simulink model "simplevector"  (R2014a)
settings: Solver=ode45  StartTime=0.0  StopTime=10.0  RelTol=1e-3
settings Model: Creator=RANGA  LastModifiedBy=RANGA

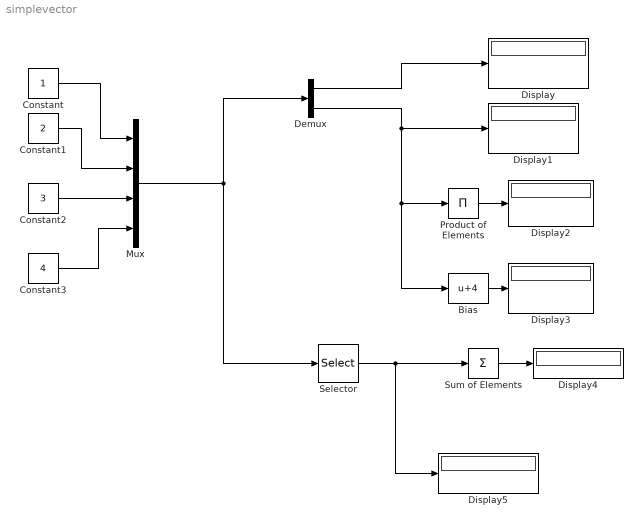
== system simplevector ==
  Bias : Bias  Bias=4
  Constant : Constant
  Constant1 : Constant  Value=2
  Constant2 : Constant  Value=3
  Constant3 : Constant  Value=4
  Demux : Demux  Outputs=2
  Display{,1..5} (6 alike) : Display
      Display settings: Decimation=2
  Mux : Mux
      settings: DisplayOption=signals
  Product of Elements : Product  Inputs=*
  Selector : Selector  InputPortWidth=4  Indices=[2 4]
  Sum of Elements : Sum  Inputs=+
  wires:
  Constant/1 -> Mux/1
  Constant1/1 -> Mux/2
  Constant2/1 -> Mux/3
  Constant3/1 -> Mux/4
  Mux/1 -> Demux/1, Selector/1
  Demux/1 -> Display/1
  Demux/2 -> Bias/1, Product of Elements/1, Display1/1
  Selector/1 -> Display5/1, Sum of Elements/1
  Bias/1 -> Display3/1
  Product of Elements/1 -> Display2/1
  Sum of Elements/1 -> Display4/1
